simulink model "CSD"  (R2020a)
settings: Solver=FixedStepAuto  StartTime=0.0  StopTime=2  RelTol=1e-3
InitFcn:
  | N = 50;
  | denfac = N*sum((0:N-1).^2)-(sum(0:N-1)).^2;
  | 
  | a2 = N/denfac;
  | a1 = sum(0:N-1)/denfac;
  | 
  | b2 = a1;
  | b1 = sum((0:N-1).^2)/denfac;
  | 
  | fs = 100e6;
  | f1 = 200e3;
undefined symbols (not defined in the file): x
settings Model: Creator=trichte  LastModifiedBy=enric
settings DataIOCC: ReturnWorkspaceOutputs=off
settings DebuggingCC: ArithmeticOperatorsInVariantConditions=warning
settings SFSimCC: SimUseLocalCustomCode=off  CustomCodeUndefinedFunction=UseInterfaceOnly
settings RTWCC: RTWUseLocalCustomCode=off

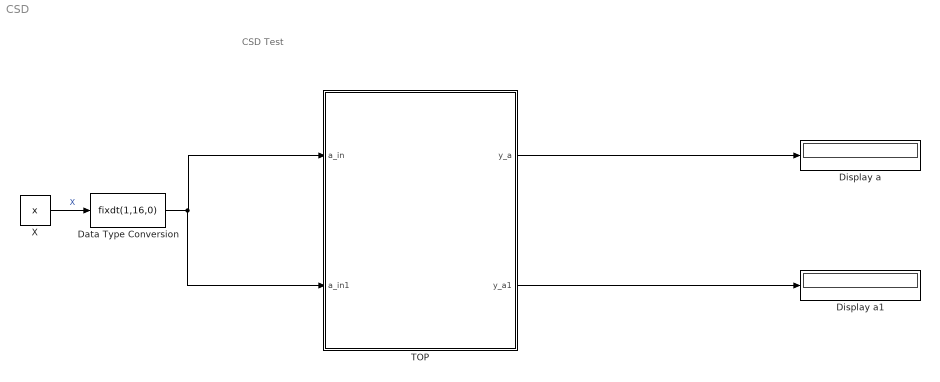
== system CSD ==
  note: CSD Test
  Data Type Conversion : DataTypeConversion  OutDataTypeStr=fixdt(1,16,0)
  Display a : Display
  Display a1 : Display
  TOP : Subsystem
  X : Constant  Value=x  OutDataTypeStr=fixdt(1,16,0)
  wires:
  TOP/1(y_a) -> Display a/1
  TOP/2(y_a1) -> Display a1/1
  X/1 -> Data Type Conversion/1  "X"
  Data Type Conversion/1 -> TOP/2(a_in1), TOP/1(a_in)

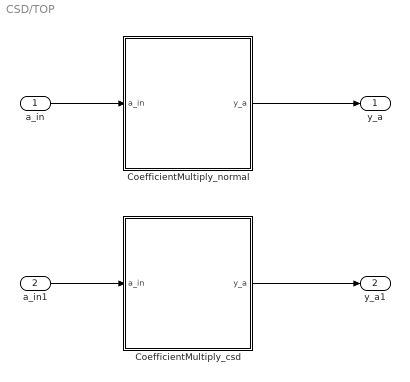
== system CSD/TOP ==
  a_in : Inport  OutDataTypeStr=fixdt(1,16,0)
  a_in1 : Inport  Port=2
  CoefficientMultiply_csd : Subsystem
  CoefficientMultiply_normal : Subsystem
  y_a : Outport  VectorParamsAs1DForOutWhenUnconnected=off
  y_a1 : Outport  Port=2  VectorParamsAs1DForOutWhenUnconnected=off
  wires:
  CoefficientMultiply_normal/1(y_a) -> y_a/1
  a_in/1 -> CoefficientMultiply_normal/1(a_in)
  a_in1/1 -> CoefficientMultiply_csd/1(a_in)
  CoefficientMultiply_csd/1(y_a) -> y_a1/1

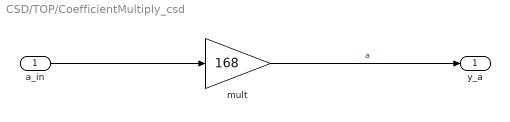
== system CSD/TOP/CoefficientMultiply_csd ==
  a_in : Inport  OutDataTypeStr=fixdt(1,16,0)
  mult : Gain  Gain=168  ParamDataTypeStr=fixdt(1,16,0)  OutDataTypeStr=fixdt(1,16,0)
  y_a : Outport  OutDataTypeStr=fixdt(1,16,0)  InitialOutput=0  VectorParamsAs1DForOutWhenUnconnected=off
  wires:
  a_in/1 -> mult/1
  mult/1 -> y_a/1  "a"

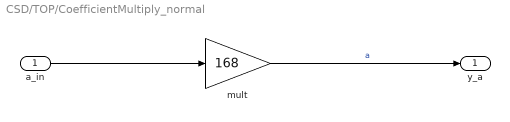
== system CSD/TOP/CoefficientMultiply_normal ==
  a_in : Inport  OutDataTypeStr=fixdt(1,16,0)
  mult : Gain  Gain=168  ParamDataTypeStr=fixdt(1,16,0)  OutDataTypeStr=fixdt(1,16,0)
  y_a : Outport  OutDataTypeStr=fixdt(1,16,0)  InitialOutput=0  VectorParamsAs1DForOutWhenUnconnected=off
  wires:
  a_in/1 -> mult/1
  mult/1 -> y_a/1  "a"
